simulink model "VMO"  (R2021a)
settings: Solver=VariableStepAuto  StartTime=0.0  StopTime=50  FixedStep=0.001  RelTol=1e-3
model workspace (MAT data in the model file):
  lambda = 0.0016
  po = [0  0  0.5; 0.5  0  0; 0  0  -0.5; -0.5  0  0]
undefined symbols (not defined in the file or in its folder): mergepose
libraries: simlib_vpc_basic x3
settings Model: Creator=marco  LastModifiedBy=marco
settings SolverCC: AlgebraicLoopSolver=TrustRegion
settings DebuggingCC: AlgebraicLoopMsg=none  SFMachineParentedDataDiag=warning
settings RTWCC: Toolchain=Clang v3.1 | gmake (64-bit Mac)

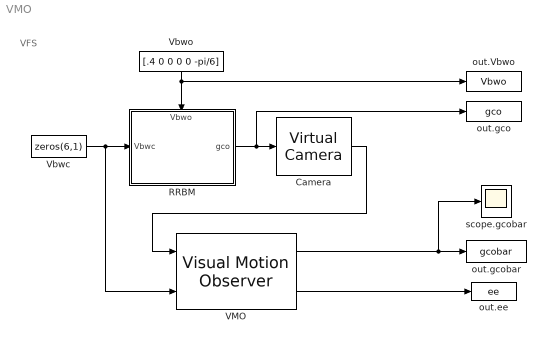
== system VMO ==
  note: VFS
  Camera : simlib_vpc_basic/Virtual Camera  camtype=Pinhole  po=po  lambda=lambda
      settings: SourceProductName=VPC Library
  RRBM : Subsystem
      settings: PortSchema="{\"entries\":[{\"content\":{\"sides\":[{\"content\":{\"connectorIds\":[\"In1\"]},\"type\":\"ConnectorPlacement.EquallySpacedRectSide\",\"uuid\":\"ce1006a6-ff18-4db7-ad69-3a60144a672f\"},{\"content\":{\"connectorIds\":[\"Out1\"],\"side\":\"RIGHT\"},\"type\":\"ConnectorPlacement.EquallySpacedRectSide\",\"uuid\":\"9f6b7cf2-eb23-4db0-862a-f9244538bf77\"},{\"content\":{\"connectorIds\":[\"In2\"],\"side\":\"TOP\"},\"type\":\"ConnectorPlacement.EquallySpacedRectSide\",\"uuid\":\"e4abfdaf-0145-4439-9abb-46234dad4713\"},{\"content\":{\"connectorIds\":[],\"side\":\"HIDDEN\"},\"type\":\"ConnectorPlacement.EquallySpacedRectSide\",\"uuid\":\"77f0040d-d5e2-4b47-95e1-996605172696\"}]},\"type\":\"ConnectorPlacement.EquallySpacedConnector\",\"uuid\":\"a30e6cf8-5cfd-45cc-9c7f-0b16cc268ba1\"}],\"packageUris\":[\"http://schema.mathworks.com/mf0/Connector/R2020b\"],\"version\":\"1.0\"}"
      mask Display:
      | % Glitch in Matlab: If you define a line whose starting point and end point
      | % is equal, then the entire mask block is plotted in bold
      | plot([0,0],[0,0])
      | 
      | % Draw Box
      | plot([0,1,1,0,0],[0,0,1,1,0])
      | 
      | % Write label
      | fprintf('1 Agent\n1 Target','texmode','on')
      | 
      | % Label ports
      | port_label('input',1,'V^{b}_{wc}','texmode','on')
      | port_label('input',2,'V^{b}_{wo}','texmode','on')
      | port_label('output',1,'g_{co}','texmode','on')
  VMO : simlib_vpc_basic/Visual Motion Observer  gcobar0=mergepose(eye(3),[0 1 0])  projection=on  Ke_source=internal  Ke=5*eye(6)  show_ue_aux=off  show_ee=on  show_dgcobar=off  camtype=Pinhole  fo=po  lambda=lambda
      settings: SourceProductName=VPC Library
  Vbwc : Constant  Value=zeros(6,1)
  Vbwo : Constant  Value=[.4 0 0 0 0 -pi/6]
  out.Vbwo : ToWorkspace  VariableName=Vbwo  SaveFormat=Structure With Time  SampleTime=-1
  out.ee : ToWorkspace  VariableName=ee  SaveFormat=Structure With Time  SampleTime=-1
  out.gco : ToWorkspace  VariableName=gco  SaveFormat=Structure With Time  SampleTime=-1
  out.gcobar : ToWorkspace  VariableName=gcobar  SaveFormat=Structure With Time  SampleTime=-1
  scope.gcobar : Scope
  wires:
  Vbwc/1 -> RRBM/1(Vbwc), VMO/2
  Vbwo/1 -> RRBM/2(Vbwo), out.Vbwo/1
  RRBM/1(gco) -> out.gco/1, Camera/1
  VMO/2 -> out.ee/1
  Camera/1 -> VMO/1
  VMO/1 -> scope.gcobar/1, out.gcobar/1

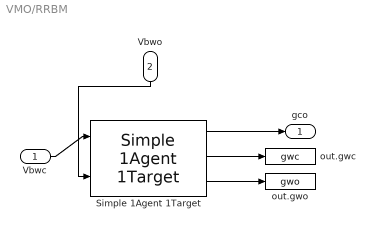
== system VMO/RRBM ==
  Vbwc : Inport
  Vbwo : Inport  Port=2
  Simple 1Agent 1Target : simlib_vpc_basic/Simple 1Agent 1Target  gwc0=mergepose(eye(3),[0 -5 0])  projectionAgent=on  gwo0=mergepose(eye(3),[0.3 0.1 0.1])  projectionTarget=on  showgwc=on  showdgwc=off  showgwo=on  showdgwo=off
      settings: SourceProductName=VPC Library
  out.gwc : ToWorkspace  VariableName=gwc  SaveFormat=Structure With Time  SampleTime=-1
  out.gwo : ToWorkspace  VariableName=gwo  SaveFormat=Structure With Time  SampleTime=-1
  gco : Outport
  wires:
  Vbwo/1 -> Simple 1Agent 1Target/2
  Vbwc/1 -> Simple 1Agent 1Target/1
  Simple 1Agent 1Target/1 -> gco/1
  Simple 1Agent 1Target/2 -> out.gwc/1
  Simple 1Agent 1Target/3 -> out.gwo/1
